simulink model "GRPSecondMotorTest"  (R2024b)
settings: Solver=VariableStepAuto  StartTime=0.0  StopTime=10.0  RelTol=1e-3
values from neighbouring files (symbols this model uses):
  h = out.yout{2}.Values.Data(:,3)    [CoefficientGradientDescent.m]    (also in DelayTime.m; SingleRunData.m)
undefined symbols (not defined in the file or in its folder): dt
libraries: simulink x2, shared6dof x2
settings Model: Creator=aniketray  LastModifiedBy=aniketray

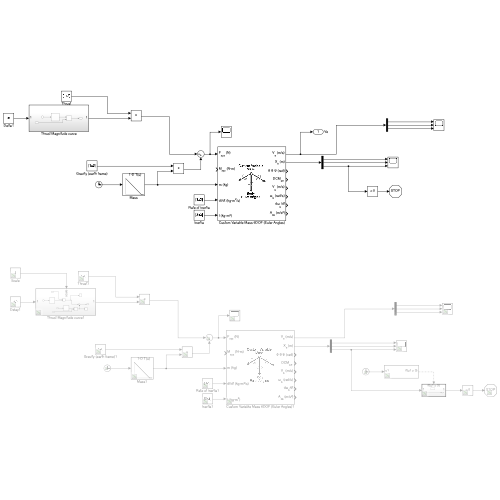
[thumbnail: Simulink's stored preview of the top-level diagram]
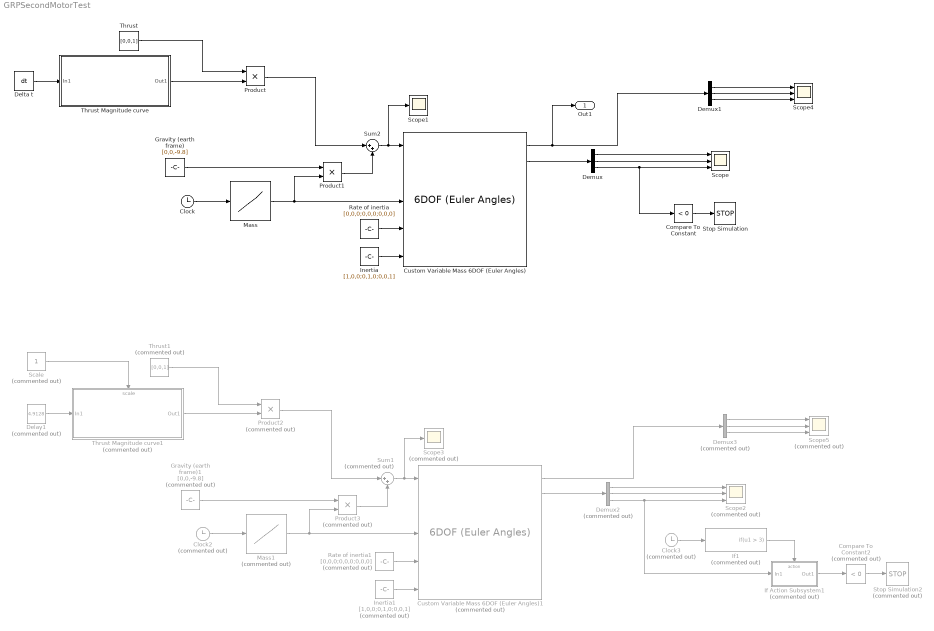
== system GRPSecondMotorTest ==
  Clock : Clock
  Clock2 : Clock  Commented=on
  Clock3 : Clock  Commented=on
  Compare To Constant : simulink/Logic and Bit Operations/Compare To Constant  relop=<  const=0  OutDataTypeStr=boolean
  Compare To Constant2 : simulink/Logic and Bit Operations/Compare To Constant  Commented=on  relop=<  const=0  OutDataTypeStr=boolean
  Custom Variable Mass 6DOF (Euler Angles) : shared6dof/6DOF (Euler Angles)  units=Metric (MKS)  mtype=Custom Variable  rep=Euler Angles  xme_0=[0 0 h]  Vm_0=[0 0 0]  eul_0=[0,0,0]  pm_0=[0 0 0]  mass_0=1.0  mass_e=0.5  mass_f=2.0  inertia=eye(3)  inertia_e=eye(3)  inertia_f=2*eye(3)  k_quat=1.0  vre_flag=off  abi_flag=off  aMode=0  xme_statename=''  Vm_statename=''  eul_statename=''  quat_statename=''  pm_statename=''  mass_statename=''
      settings: LibrarySourceBlock=aerolib6dof2/Custom Variable Mass 6DOF (Euler Angles)
  Custom Variable Mass 6DOF (Euler Angles)1 : shared6dof/6DOF (Euler Angles)  Commented=on  units=Metric (MKS)  mtype=Custom Variable  rep=Euler Angles  xme_0=[0 0 0]  Vm_0=[0 0 0]  eul_0=[0,0,0]  pm_0=[0 0 0]  mass_0=1.0  mass_e=0.5  mass_f=2.0  inertia=eye(3)  inertia_e=eye(3)  inertia_f=2*eye(3)  k_quat=1.0  vre_flag=off  abi_flag=off  aMode=0  xme_statename=''  Vm_statename=''  eul_statename=''  quat_statename=''  pm_statename=''  mass_statename=''
      settings: LibrarySourceBlock=aerolib6dof2/Custom Variable Mass 6DOF (Euler Angles)
  Delay1 : Constant  Commented=on  Value=4.9128
  Delta t : Constant  Value=dt
  Demux : Demux  Outputs=3
  Demux1 : Demux  Outputs=3
  Demux2 : Demux  Commented=on  Outputs=3
  Demux3 : Demux  Commented=on  Outputs=3
  Gravity (earth frame) : Constant  Value=[0,0,-9.8]
  Gravity (earth frame)1 : Constant  Commented=on  Value=[0,0,-9.8]
  If Action Subsystem1 : Subsystem  Commented=on  TreatAsAtomicUnit=on
  If1 : If  Commented=on  IfExpression=u1 > 3  ShowElse=off
  Inertia : Constant  Value=[1,0,0;0,1,0;0,0,1]
  Inertia1 : Constant  Commented=on  Value=[1,0,0;0,1,0;0,0,1]
  Mass : Lookup_n-D  NumberOfTableDimensions=1  BreakpointsForDimension1=[0,3.45, 4]  Table=[1.2+0.06,1.2, 1.2]  InternalRulePriority=Speed  RndMeth=Simplest
  Mass1 : Lookup_n-D  Commented=on  NumberOfTableDimensions=1  BreakpointsForDimension1=[0,3.45, 4]  Table=[1.2+0.06,1.2, 1.2]  InternalRulePriority=Speed  RndMeth=Simplest
  Product : Product
  Product1 : Product
  Product2 : Product  Commented=on
  Product3 : Product  Commented=on
  Rate of inertia : Constant  Value=[0,0,0;0,0,0;0,0,0]
  Rate of inertia1 : Constant  Commented=on  Value=[0,0,0;0,0,0;0,0,0]
  Scale : Constant  Commented=on
  Scope : Scope  NumInputPorts=3
  Scope1 : Scope
  Scope2 : Scope  Commented=on  NumInputPorts=3
  Scope3 : Scope  Commented=on
  Scope4 : Scope  NumInputPorts=3
  Scope5 : Scope  Commented=on  NumInputPorts=3
  Stop Simulation : Stop
  Stop Simulation2 : Stop  Commented=on
  Sum1 : Sum  Commented=on  Inputs=|++
  Sum2 : Sum  Inputs=|++
  Thrust : Constant  Value=[0,0,1]
  Thrust Magnitude curve : Subsystem
  Thrust Magnitude curve1 : Subsystem  Commented=on
      settings: PortSchema="{\"entries\":[{\"content\":{\"sides\":[{\"content\":{\"connectorIds\":[\"In1\"]},\"type\":\"ConnectorPlacement.EquallySpacedRectSide\",\"uuid\":\"6c79749f-0911-4e99-bba1-fa3928c950b8\"},{\"content\":{\"connectorIds\":[\"Out1\"],\"side\":\"RIGHT\"},\"type\":\"ConnectorPlacement.EquallySpacedRectSide\",\"uuid\":\"ea679260-2055-4b09-b264-5d8f9c786318\"},{\"content\":{\"connectorIds\":[\"In2\"],\"side\":\"TOP\"},\"type\":\"ConnectorPlacement.EquallySpacedRectSide\",\"uuid\":\"5d419add-cef8-4317-8c87-04a8d4eb9ead\"}]},\"type\":\"ConnectorPlacement.EquallySpacedConnector\",\"uuid\":\"9eb34e48-0e08-468e-a7c4-c098aec96b82\"}],\"packageUris\":[\"http://schema.mathworks.com/mf0/Connector/R2020b\"],\"version\":\"1.0\"}"
  Thrust1 : Constant  Commented=on  Value=[0,0,1]
  Out1 : Outport  SignalName=Ve
  wires:
  Clock/1 -> Mass/1
  Mass/1 -> Custom Variable Mass 6DOF (Euler Angles)/3, Product1/2
  Gravity (earth frame)/1 -> Product1/1
  Product1/1 -> Sum2/2
  Delta t/1 -> Thrust Magnitude curve/1(In1)
  Thrust/1 -> Product/1
  Sum2/1 -> Scope1/1, Custom Variable Mass 6DOF (Euler Angles)/1
  Demux/2 -> Scope/2
  Demux/1 -> Scope/1
  Compare To Constant/1 -> Stop Simulation/1
  Custom Variable Mass 6DOF (Euler Angles)/2 -> Demux/1
  Demux/3 -> Compare To Constant/1, Scope/3
  Inertia/1 -> Custom Variable Mass 6DOF (Euler Angles)/5
  Rate of inertia/1 -> Custom Variable Mass 6DOF (Euler Angles)/4
  Demux1/1 -> Scope4/1
  Demux1/2 -> Scope4/2
  Demux1/3 -> Scope4/3
  Custom Variable Mass 6DOF (Euler Angles)/1 -> Out1/1, Demux1/1
  Delay1/1 -> Thrust Magnitude curve1/1(In1)
  Product/1 -> Sum2/1
  Scale/1 -> Thrust Magnitude curve1/2(scale)
  Thrust Magnitude curve/1(Out1) -> Product/2
  Demux3/2 -> Scope5/2
  Demux3/1 -> Scope5/1
  Rate of inertia1/1 -> Custom Variable Mass 6DOF (Euler Angles)1/4
  If Action Subsystem1/1(Out1) -> Compare To Constant2/1
  Demux3/3 -> Scope5/3
  Thrust1/1 -> Product2/1
  Clock2/1 -> Mass1/1
  Gravity (earth frame)1/1 -> Product3/1
  Demux2/3 -> If Action Subsystem1/1(In1), Scope2/3
  Demux2/2 -> Scope2/2
  Product3/1 -> Sum1/2
  Custom Variable Mass 6DOF (Euler Angles)1/2 -> Demux2/1
  Mass1/1 -> Custom Variable Mass 6DOF (Euler Angles)1/3, Product3/2
  Product2/1 -> Sum1/1
  Compare To Constant2/1 -> Stop Simulation2/1
  Inertia1/1 -> Custom Variable Mass 6DOF (Euler Angles)1/5
  If1/1 -> If Action Subsystem1/Action
  Custom Variable Mass 6DOF (Euler Angles)1/1 -> Demux3/1
  Clock3/1 -> If1/1
  Thrust Magnitude curve1/1(Out1) -> Product2/2
  Sum1/1 -> Scope3/1, Custom Variable Mass 6DOF (Euler Angles)1/1
  Demux2/1 -> Scope2/1

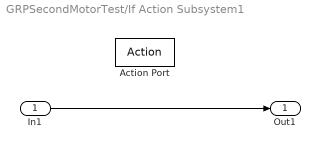
== system GRPSecondMotorTest/If Action Subsystem1 ==
  In1 : Inport
  Action Port : ActionPort  ActionPortLabel=if(u1 > 3)
  Out1 : Outport
  wires:
  In1/1 -> Out1/1

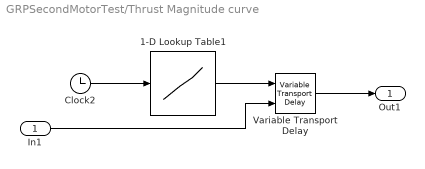
== system GRPSecondMotorTest/Thrust Magnitude curve ==
  In1 : Inport
  1-D Lookup Table1 : Lookup_n-D  NumberOfTableDimensions=1  BreakpointsForDimension1=[-10;0;0.063;0.11799999999999999;0.158;0.22800000000000001;0.34000000000000002;0.38600000000000001;0.42499999999999999;0.48099999999999998;0.58299999999999996;0.88300000000000001;1.1910000000000001;1.3640000000000001;1.569;1.7270000000000001;2;2.3900000000000001;2.6800000000000002;2.96;3.25;3.3500000000000001;3.3900000000000001;3.3999999999999999;10]  Table=[0;0;2.1269999999999998;4.407;8.359;13.68;20.82;26.75;25.379999999999999;22.190000000000001;17.93;16.109999999999999;14.59;15.35;15.65;14.74;14.279999999999999;13.68;13.08;13.07;13.050000000000001;13;7.2999999999999998;0;0]  InternalRulePriority=Speed  RndMeth=Simplest
  Clock2 : Clock
  Variable Transport Delay : VariableTransportDelay  VariableDelayType=Variable transport delay  MaximumDelay=6  TransDelayFeedthrough=on
  Out1 : Outport
  wires:
  In1/1 -> Variable Transport Delay/2
  1-D Lookup Table1/1 -> Variable Transport Delay/1
  Variable Transport Delay/1 -> Out1/1
  Clock2/1 -> 1-D Lookup Table1/1

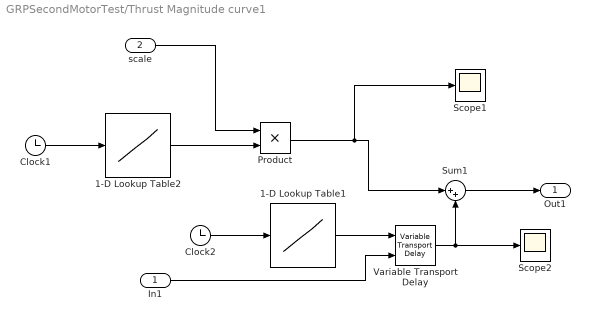
== system GRPSecondMotorTest/Thrust Magnitude curve1 ==
  In1 : Inport
  scale : Inport  Port=2
  1-D Lookup Table1 : Lookup_n-D  NumberOfTableDimensions=1  BreakpointsForDimension1=[-10;0;0.063;0.11799999999999999;0.158;0.22800000000000001;0.34000000000000002;0.38600000000000001;0.42499999999999999;0.48099999999999998;0.58299999999999996;0.88300000000000001;1.1910000000000001;1.3640000000000001;1.569;1.7270000000000001;2;2.3900000000000001;2.6800000000000002;2.96;3.25;3.3500000000000001;3.3900000000000001;3.3999999999999999;10]  Table=[0;0;2.1269999999999998;4.407;8.359;13.68;20.82;26.75;25.379999999999999;22.190000000000001;17.93;16.109999999999999;14.59;15.35;15.65;14.74;14.279999999999999;13.68;13.08;13.07;13.050000000000001;13;7.2999999999999998;0;0]  InternalRulePriority=Speed  RndMeth=Simplest
  1-D Lookup Table2 : Lookup_n-D  NumberOfTableDimensions=1  BreakpointsForDimension1=[0;0.063;0.11799999999999999;0.158;0.22800000000000001;0.34000000000000002;0.38600000000000001;0.42499999999999999;0.48099999999999998;0.58299999999999996;0.88300000000000001;1.1910000000000001;1.3640000000000001;1.569;1.7270000000000001;2;2.3900000000000001;2.6800000000000002;2.96;3.25;3.3500000000000001;3.3900000000000001;3.3999999999999999;10]  Table=[0;2.1269999999999998;4.407;8.359;13.68;20.82;26.75;25.379999999999999;22.190000000000001;17.93;16.109999999999999;14.59;15.35;15.65;14.74;14.279999999999999;13.68;13.08;13.07;13.050000000000001;13;7.2999999999999998;0;0]  InternalRulePriority=Speed  RndMeth=Simplest
  Clock1 : Clock
  Clock2 : Clock
  Product : Product
  Scope1 : Scope
  Scope2 : Scope
  Sum1 : Sum  Inputs=|++
  Variable Transport Delay : VariableTransportDelay  VariableDelayType=Variable transport delay  MaximumDelay=6  TransDelayFeedthrough=on
  Out1 : Outport
  wires:
  In1/1 -> Variable Transport Delay/2
  Clock1/1 -> 1-D Lookup Table2/1
  Variable Transport Delay/1 -> Sum1/2, Scope2/1
  1-D Lookup Table1/1 -> Variable Transport Delay/1
  Sum1/1 -> Out1/1
  Clock2/1 -> 1-D Lookup Table1/1
  1-D Lookup Table2/1 -> Product/2
  scale/1 -> Product/1
  Product/1 -> Scope1/1, Sum1/1
